simulink model "TVCLaunch"  (R2024b)
settings: Solver=VariableStepAuto  StartTime=0.0  StopTime=30  FixedStep=0.0001  MaxStep=0.0001  RelTol=1e-3
model workspace (MAT data in the model file):
  Mass = 0.5
undefined symbols (not defined in the file): DiscIntNeverNeededParam
libraries: simulink x3, simulink_extras x2, slpidlib x2, dspfdesign x1
settings Model: Creator=jebid  LastModifiedBy=jebid

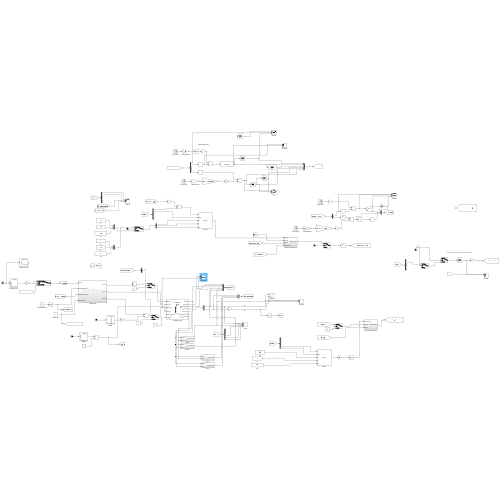
[thumbnail: Simulink's stored preview of the top-level diagram]
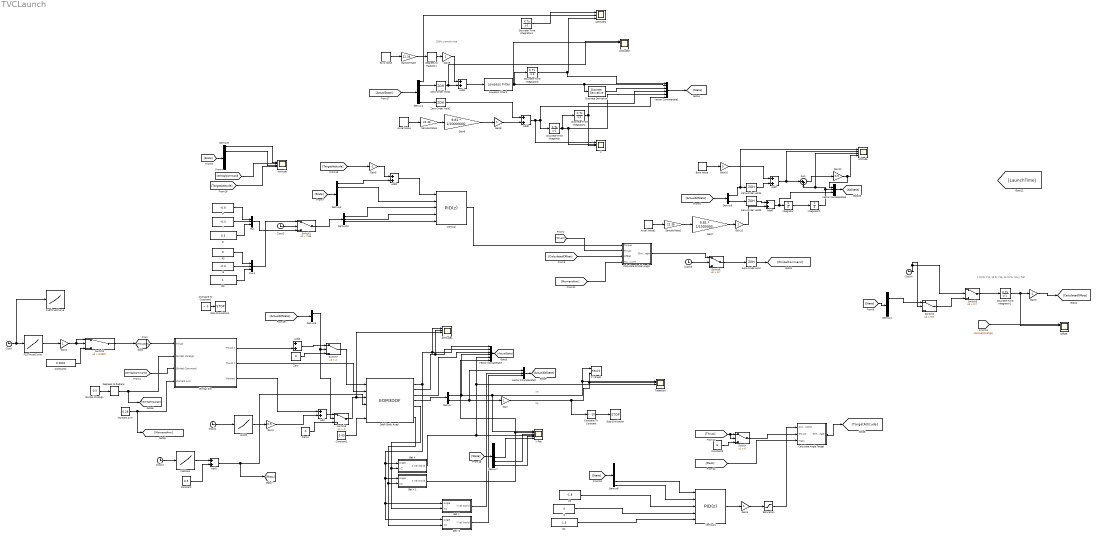
== system TVCLaunch ==
  note: 250hz sample rate
  note: 1.19 for F10, 18 for F15, 23.75 for noisy f15?
  note: Ze
  note: Xe
  3dof (Body Axes) : EOM3DOF  mtype=Custom Variable  v_ini=0  theta_ini=0.09  mass=0.5  Iyy=0.05  g=-9.81  abi_flag=on
  Accel Noise : RandomNumber  Variance=70  SampleTime=0.002
  Accel Noise1 : RandomNumber  Variance=70  SampleTime=0.002
  Add{,1..7} (8 alike) : Sum
  Altitude : Scope  NumInputPorts=5
  Attitude{,1..2,4} (4 alike) : Scope  NumInputPorts=5
  BUMP : Lookup_n-D  NumberOfTableDimensions=1  BreakpointsForDimension1=[-5 -4 -3 -2 -1 0 1 1.1000000000000001 1.2 1.3 5]  Table=[0 0 0 0 0 0 0 0.28000000000000003 0.28000000000000003 0 0]  InternalRulePriority=Speed  RndMeth=Simplest
  Baro Noise : RandomNumber  Variance=0.1  SampleTime=0.002
  Calculate Angle Target : Subsystem
  Calculate Gimbal Angle : Subsystem
  Clock{,1..2,4..6} (6 alike) : Clock
  Compare To Constant : simulink/Logic and Bit Operations/Compare To Constant  relop=<  const=-10  OutDataTypeStr=boolean
  Compare To Constant1 : simulink/Logic and Bit Operations/Compare To Constant  relop=<  const=0  OutDataTypeStr=boolean
  Constant : Constant  Value=0.5
  Constant1 : Constant  Value=0.05
  Constant2 : Constant  Value=0.0001
  Constant3 : Constant  Value=6
  D : Constant  Value=0.3
  D2 : Constant  Value=1.5
  D3 : Constant
  Degrees to Radians : simulink_extras/Transformations/Degrees to Radians
  Degrees to Radians1 : simulink_extras/Transformations/Degrees to Radians
  Demux : Demux  Outputs=2
  Demux{1,3..7} (6 alike) : Demux  Outputs=6
  Demux10 : Demux  Outputs=3
  Demux8 : Demux  Outputs=3
  Demux9 : Demux  Outputs=3
  Discrete Derivative : simulink/Discrete/Discrete Derivative  gainval=1.0  ICPrevScaledInput=0.0  OutMin=[]  OutMax=[]  OutDataType=fixdt(1, 16)  OutScaling=2^-10  DoSatur=off
  Discrete-Time Integrator : DiscreteIntegrator  SampleTime=0.01  ICPrevOutput=DiscIntNeverNeededParam  ICPrevScaledInput=DiscIntNeverNeededParam
  Discrete-Time Integrator1 : DiscreteIntegrator  gainval=20  SampleTime=0.01  ICPrevOutput=DiscIntNeverNeededParam  ICPrevScaledInput=DiscIntNeverNeededParam
  Discrete-Time Integrator2 : DiscreteIntegrator  SampleTime=0.01  ICPrevOutput=DiscIntNeverNeededParam  ICPrevScaledInput=DiscIntNeverNeededParam
  Discrete-Time Integrator3 : DiscreteIntegrator  InitialCondition=0.09  SampleTime=0.01  ICPrevOutput=DiscIntNeverNeededParam  ICPrevScaledInput=DiscIntNeverNeededParam
  Discrete-Time Integrator4 : DiscreteIntegrator  SampleTime=0.01  ICPrevOutput=DiscIntNeverNeededParam  ICPrevScaledInput=DiscIntNeverNeededParam
  F10ThrustCurve : Lookup_n-D  NumberOfTableDimensions=1  BreakpointsForDimension1=[0.015;0.077;0.201;0.31;0.464;0.573;0.789;1.068;1.393;1.718;2.166;2.677;3.311;3.683;3.791;4.101;4.658;5.168;5.725;6.112;6.329;6.499;6.685;6.778;6.917;7.025;7.13]  Table=[28.22;26.082;24.934;22.806;20.183;17.886;16.075;13.946;12.63;11.155;9.843999999999999;9.515000000000001;9.186999999999999;8.859;9.679;9.679;9.515000000000001;9.023;9.023;8.531000000000001;8.859;7.546;5.742;4.921;2.625;1.312;-0.001]  InternalRulePriority=Speed  RndMeth=Simplest
  F15Mass : Lookup_n-D  NumberOfTableDimensions=1  BreakpointsForDimension1=[0;0.14799999999999999;0.22800000000000001;0.29399999999999998;0.35299999999999998;0.38200000000000001;0.41899999999999998;0.47699999999999998;0.52000000000000002;0.59299999999999997;0.68799999999999994;0.85499999999999998;1.0369999999999999;1.2050000000000001;1.423;1.452;1.5029999999999999;1.736;1.9550000000000001;2.21;2.4940000000000002;2.7629999999999999;3.1200000000000001;3.3820000000000001;3.4039999999999999;3.4180000000000001;3.4500000000000002;60]  Table=[0.102;0.101316;0.100354;0.09921099999999999;0.09790500000000001;0.097151;0.096077;0.09438199999999999;0.09324;0.091477;0.089374;0.085969;0.082485;0.079399;0.0755;0.07496700000000001;0.07402599999999999;0.069882;0.066051;0.061665;0.056863;0.052445;0.046687;0.042513;0.042215;0.042095;0.042;0.042]  InternalRulePriority=Speed  RndMeth=Simplest
  F15ThrustCurve : Lookup_n-D  NumberOfTableDimensions=1  BreakpointsForDimension1=[0;0.14799999999999999;0.22800000000000001;0.29399999999999998;0.35299999999999998;0.38200000000000001;0.41899999999999998;0.47699999999999998;0.52000000000000002;0.59299999999999997;0.68799999999999994;0.85499999999999998;1.0369999999999999;1.2050000000000001;1.423;1.452;1.5029999999999999;1.736;1.9550000000000001;2.21;2.4940000000000002;2.7629999999999999;3.1200000000000001;3.3820000000000001;3.4039999999999999;3.4180000000000001;3.4500000000000002;60]  Table=[0;7.6379999999999999;12.253;16.390999999999998;20.210000000000001;22.756;25.260000000000002;23.074000000000002;20.844999999999999;19.093;17.5;16.225000000000001;15.427;14.948;14.627000000000001;15.741;14.785;14.622999999999999;14.303000000000001;14.141;13.819000000000001;13.337999999999999;13.334;13.013;9.3520000000000003;4.8949999999999996;-0.001;-0.001]  InternalRulePriority=Speed  RndMeth=Simplest
  Gain{,2,4,8..9,11} (6 alike) : Gain
  Gain1 : Gain  Gain=0.5
  Gain10 : Gain  Gain=5
  Gain12 : Gain  Gain=0.5
  Gain3 : Gain  Gain=-1
  Gain5 : Gain  Gain=-1
  Gain6 : Gain  Gain=9.81 * 1/10000000
  Gain7 : Gain  Gain=9.81 * 1/1000000
  Get X : Subsystem
  Get X 1 : Subsystem
  Get Y : Subsystem
  Get Y1 : Subsystem
  Gimbal Misalign : Constant  Value=0.5
  Gimbal Sim : Subsystem
  Gyro Noise : RandomNumber  Variance=0.0028  SampleTime=0.002
  I : Constant  Value=-0.3  VectorParams1D=off
  I2 : Constant  Value=0  VectorParams1D=off
  I3 : Constant  Value=-0.3  VectorParams1D=off
  Integrator : Integrator
  Integrator1 : Integrator
  Lowpass Filter1 : dspfdesign/Lowpass Filter  FilterType=IIR  DesignForMinimumOrder=on  FilterOrder=50  PassbandFrequency=7.5  StopbandFrequency=247.5  PassbandRipple=0.1  StopbandAttenuation=100  SampleRateMode=Specify on dialog  SampleRate=500  SimulateUsing=Interpreted execution  roundingMode=Floor  coeffsDataTypeStr=fixdt(1,16)
  Moment Arm : Constant  Value=0.28
  Mux : Mux  Inputs=3
  Mux1 : Mux  Inputs=3
  Offset : Scope  NumInputPorts=5
  P : Constant  Value=-0.9
  P2 : Constant  Value=-1.8
  P3 : Constant  Value=0
  Sample Rate : Gain  Gain=22.36
  Sample Rate1 : Gain  Gain=22.36
  Sample Rate2 : Gain  Gain=22.36
  Saturation : Saturate  UpperLimit=8  LowerLimit=-8
  Stop Simulation : Stop
  Stop Simulation1 : Stop
  Sum : Sum  Inputs=|++
  Switch : Switch  Criteria=u2 > Threshold  Threshold=6  SaturateOnIntegerOverflow=off  InputSameDT=off
  Switch1 : Switch  Criteria=u2 > Threshold  Threshold=2.85  SaturateOnIntegerOverflow=off  InputSameDT=off
  Switch2 : Switch  Criteria=u2 > Threshold  Threshold=0.6  SaturateOnIntegerOverflow=off  InputSameDT=off
  Switch3 : Switch  Criteria=u2 > Threshold  Threshold=0.7  SaturateOnIntegerOverflow=off  InputSameDT=off
  Switch4 : Switch  Criteria=u2 > Threshold  Threshold=0.0001  SaturateOnIntegerOverflow=off  InputSameDT=off
  Switch6 : Switch  Criteria=u2 > Threshold  Threshold=0.7  SaturateOnIntegerOverflow=off  InputSameDT=off
  Switch7 : Switch  Criteria=u2 > Threshold  Threshold=2  SaturateOnIntegerOverflow=off  InputSameDT=off
  Switch8 : Switch  Criteria=u2 > Threshold  Threshold=2  SaturateOnIntegerOverflow=off  InputSameDT=off
  Trajectory : Scope  NumInputPorts=5
  Vector Concatenate : Concatenate  NumInputs=6
  Vector Concatenate1 : Concatenate  NumInputs=6
  Vector Concatenate2 : Concatenate  NumInputs=3
  Vector Concatenate3 : Concatenate  NumInputs=3
  Vertical : slpidlib/PID Controller  Controller=PID  Form=Parallel  TimeDomain=Discrete-time  UseExternalTs=off  SampleTime=0.01  IntegratorMethod=Forward Euler  FilterMethod=Forward Euler  ControllerParametersSource=external  P=1  I=1  UseKiTs=off  D=0  UseExternalDerivativeSource=on  N=100  UseFilter=off  TunerSelectOption=Transfer Function Based (PID Tuner App)  InitialConditionSource=internal  InitialConditionForIntegrator=0  InitialConditionForFilter=0  DifferentiatorICPrevScaledInput=0  ExternalReset=none  TrackingMode=off  Kt=1  LimitOutput=off  SatLimitsSource=internal  UpperSaturationLimit=inf  LowerSaturationLimit=-inf  LinearizeAsGain=off  AntiWindupMode=none  Kb=1  LimitIntegrator=off  UpperIntegratorSaturationLimit=inf  LowerIntegratorSaturationLimit=-inf  POutMin=[]  POutMax=[]  IOutMin=[]  IOutMax=[]  DOutMin=[]  DOutMax=[]  NOutMin=[]  NOutMax=[]  SumOutMin=[]  SumOutMax=[]  SaturationOutMin=[]  SaturationOutMax=[]  PParamMin=[]  PParamMax=[]  IParamMin=[]  IParamMax=[]  DParamMin=[]  DParamMax=[]  NParamMin=[]  NParamMax=[]  KbParamMin=[]  KbParamMax=[]  KtParamMin=[]  KtParamMax=[]  KbOutMin=[]  KbOutMax=[]  KtOutMin=[]  KtOutMax=[]  IntegratorOutMin=[]  IntegratorOutMax=[]  FilterOutMin=[]  FilterOutMax=[]  SumI1OutMin=[]  SumI1OutMax=[]  SumI2OutMin=[]  SumI2OutMax=[]  SumI3OutMin=[]  SumI3OutMax=[]  SumI4OutMin=[]  SumI4OutMax=[]  SumDOutMin=[]  SumDOutMax=[]  DifferentiatorOutMin=[]  DifferentiatorOutMax=[]  FilterDiffOutCoefMin=[]  FilterDiffOutCoefMax=[]  ReciprocalOutMin=[]  ReciprocalOutMax=[]  SumDenOutMin=[]  SumDenOutMax=[]  SumNumOutMin=[]  SumNumOutMax=[]  DivideOutMin=[]  DivideOutMax=[]  UdiffTsProdOutMin=[]  UdiffTsProdOutMax=[]  NTsProdOutMin=[]  NTsProdOutMax=[]  UintegralTsProdOutMin=[]  UintegralTsProdOutMax=[]  UngainTsProdOutMin=[]  UngainTsProdOutMax=[]  ClampingZeroOutDataTypeStr=Inherit: Inherit via back propagation  ClampingZeroOutMin=[]  ClampingZeroOutMax=[]  FilterDenConstantOutDataTypeStr=Inherit: Inherit via back propagation  FilterDenConstantOutMin=[]  FilterDenConstantOutMax=[]  PCopyOutDataTypeStr=Inherit: Inherit via back propagation  PCopyOutMin=[]  PCopyOutMax=[]  NCopyOutDataTypeStr=Inherit: Inherit via back propagation  NCopyOutMin=[]  NCopyOutMax=[]  IntegratorContinuousStateAttributes=''  IntegratorStateMustResolveToSignalObject=off  IntegratorRTWStateStorageClass=Auto  FilterContinuousStateAttributes=''  FilterStateMustResolveToSignalObject=off  FilterRTWStateStorageClass=Auto  ParallelPVariant=ExternalParameters  IdealPVariant=Disabled  IVariant=ExternalParameters  DVariant=ExternalParameters  IntegratorVariant=Discrete  SatVariant=Disabled  AWVariant=Passthrough  PCopyVariant=Disabled  TRVariant=Disabled  FdbkBlocksVariant=Forward  IdealPFdbkVariant=Disabled  SatFdbkVariant=Disabled  DerivativeFilterVariant=Passthrough  NVariant=Passthrough  NCopyVariant=Disabled_SignalSpec  FilterICVariant=Disabled  IntegratorICVariant=InternalICs  ExternalResetVariant=Disabled  TRSumVariant=Passthrough  SumFdbkVariant=Disabled  SumVariant=Sum_PID  TsampFilterVariant=InternalTs  TsampNgainVariant=Passthrough  TsampIntegralVariant=Disabled_SignalSpec  ExternalSaturationOutDataTypeStr=Inherit: Same as second input  DerivativeSourceVariant=ExternalYdot  PreIntVariant=InternalPreInt
      settings: LibrarySourceBlock=simulink/Discrete/Discrete PID Controller
  Vertical1 : slpidlib/PID Controller  Controller=PID  Form=Parallel  TimeDomain=Discrete-time  UseExternalTs=off  SampleTime=0.01  IntegratorMethod=Forward Euler  FilterMethod=Forward Euler  ControllerParametersSource=external  P=1  I=1  UseKiTs=off  D=0  UseExternalDerivativeSource=on  N=100  UseFilter=off  TunerSelectOption=Transfer Function Based (PID Tuner App)  InitialConditionSource=internal  InitialConditionForIntegrator=0  InitialConditionForFilter=0  DifferentiatorICPrevScaledInput=0  ExternalReset=none  TrackingMode=off  Kt=1  LimitOutput=off  SatLimitsSource=internal  UpperSaturationLimit=inf  LowerSaturationLimit=-inf  LinearizeAsGain=off  AntiWindupMode=none  Kb=1  LimitIntegrator=off  UpperIntegratorSaturationLimit=inf  LowerIntegratorSaturationLimit=-inf  POutMin=[]  POutMax=[]  IOutMin=[]  IOutMax=[]  DOutMin=[]  DOutMax=[]  NOutMin=[]  NOutMax=[]  SumOutMin=[]  SumOutMax=[]  SaturationOutMin=[]  SaturationOutMax=[]  PParamMin=[]  PParamMax=[]  IParamMin=[]  IParamMax=[]  DParamMin=[]  DParamMax=[]  NParamMin=[]  NParamMax=[]  KbParamMin=[]  KbParamMax=[]  KtParamMin=[]  KtParamMax=[]  KbOutMin=[]  KbOutMax=[]  KtOutMin=[]  KtOutMax=[]  IntegratorOutMin=[]  IntegratorOutMax=[]  FilterOutMin=[]  FilterOutMax=[]  SumI1OutMin=[]  SumI1OutMax=[]  SumI2OutMin=[]  SumI2OutMax=[]  SumI3OutMin=[]  SumI3OutMax=[]  SumI4OutMin=[]  SumI4OutMax=[]  SumDOutMin=[]  SumDOutMax=[]  DifferentiatorOutMin=[]  DifferentiatorOutMax=[]  FilterDiffOutCoefMin=[]  FilterDiffOutCoefMax=[]  ReciprocalOutMin=[]  ReciprocalOutMax=[]  SumDenOutMin=[]  SumDenOutMax=[]  SumNumOutMin=[]  SumNumOutMax=[]  DivideOutMin=[]  DivideOutMax=[]  UdiffTsProdOutMin=[]  UdiffTsProdOutMax=[]  NTsProdOutMin=[]  NTsProdOutMax=[]  UintegralTsProdOutMin=[]  UintegralTsProdOutMax=[]  UngainTsProdOutMin=[]  UngainTsProdOutMax=[]  ClampingZeroOutDataTypeStr=Inherit: Inherit via back propagation  ClampingZeroOutMin=[]  ClampingZeroOutMax=[]  FilterDenConstantOutDataTypeStr=Inherit: Inherit via back propagation  FilterDenConstantOutMin=[]  FilterDenConstantOutMax=[]  PCopyOutDataTypeStr=Inherit: Inherit via back propagation  PCopyOutMin=[]  PCopyOutMax=[]  NCopyOutDataTypeStr=Inherit: Inherit via back propagation  NCopyOutMin=[]  NCopyOutMax=[]  IntegratorContinuousStateAttributes=''  IntegratorStateMustResolveToSignalObject=off  IntegratorRTWStateStorageClass=Auto  FilterContinuousStateAttributes=''  FilterStateMustResolveToSignalObject=off  FilterRTWStateStorageClass=Auto  ParallelPVariant=ExternalParameters  IdealPVariant=Disabled  IVariant=ExternalParameters  DVariant=ExternalParameters  IntegratorVariant=Discrete  SatVariant=Disabled  AWVariant=Passthrough  PCopyVariant=Disabled  TRVariant=Disabled  FdbkBlocksVariant=Forward  IdealPFdbkVariant=Disabled  SatFdbkVariant=Disabled  DerivativeFilterVariant=Passthrough  NVariant=Passthrough  NCopyVariant=Disabled_SignalSpec  FilterICVariant=Disabled  IntegratorICVariant=InternalICs  ExternalResetVariant=Disabled  TRSumVariant=Passthrough  SumFdbkVariant=Disabled  SumVariant=Sum_PID  TsampFilterVariant=InternalTs  TsampNgainVariant=Passthrough  TsampIntegralVariant=Disabled_SignalSpec  ExternalSaturationOutDataTypeStr=Inherit: Same as second input  DerivativeSourceVariant=ExternalYdot  PreIntVariant=InternalPreInt
      settings: LibrarySourceBlock=simulink/Discrete/Discrete PID Controller
  X : Scope  NumInputPorts=5
  X Pos : Scope  NumInputPorts=6
  XY Graph : Record  FileSettingsInternal="{\"entries\":[{\"content\":{\"excelSettings\":{\"content\":{},\"type\":\"Streamout.ExcelSettings\"}},\"type\":\"Streamout.FileSettingStorage\",\"uuid\":\"\"}],\"packageUris\":[\"http:\\/\\/schema.mathworks.com\\/mf0\\/streamout_blocks\\/R2020a\"],\"version\":\"1.0\"}"  Layout=[1 1]  SignalsInternal="{\"entries\":[{\"content\":{\"signals\":[{\"content\":{\"blockPath\":[],\"dimensions\":[1],\"domain\":\"\",\"lineColor\":\"#a2142f\",\"plots\":[ 1 ],\"port\":1,\"sid\":[\"\"],\"signalID\":1,\"signalName\":\"Demux:1\"},\"type\":\"RecordBlkView.Signal\",\"uuid\":\"\"},{\"content\":{\"blockPath\":[],\"dimensions\":[1],\"domain\":\"\",\"lineColor\":\"#139fff\",\"plots\":[ 1 ],\"port\":2,\"sid\":[\"\"],\"signalID\":2,\"signalName\":\"Gain\"},\"type\":\"RecordBlkView.Signal\",\"uuid\":\"\"}]},\"type\":\"RecordBlkView.InputSignals\",\"uuid\":\"\"}],\"packageUris\":[\"http:\\/\\/schema.mathworks.com\\/mf0\\/streamout_blocks\\/R2020a\"],\"version\":\"1.0\"}"  VisualizationBindings="{\"xyplotplugin\":{\"info\":[{\"series\":[{\"bindingParametersList\":[{\"parameter\":\"X-Axis\",\"signalID\":1,\"signalName\":\"Demux:1\"},{\"parameter\":\"Y-Axis\",\"signalID\":2,\"signalName\":\"Gain\"}],\"seriesID\":0}],\"subplotID\":1}]}}"  CompatibilityTag=XY
  Zero : Constant  Value=0  OutDataTypeStr=Inherit: Inherit via back propagation
  Zero-Order Hold : ZeroOrderHold  SampleTime=0.02
  Zero-Order Hold{1..4} (4 alike) : ZeroOrderHold  SampleTime=0.002
  Zero1 : Constant  Value=0  OutDataTypeStr=Inherit: Inherit via back propagation
  wires:
  3dof (Body Axes)/4 -> Demux/1
  Demux/2 -> Vector Concatenate2/1, Gain/1
  Gain/1 -> Compare To Constant/1, XY Graph/2, Trajectory/2
  Clock/1 -> F10ThrustCurve/1, F15ThrustCurve/1
  Compare To Constant/1 -> Stop Simulation/1
  Gimbal Misalign/1 -> Degrees to Radians/1
  Moment Arm/1 -> [MomentArm], Gimbal Sim/4(Moment Arm)
  3dof (Body Axes)/1 -> Get Y1/1(Angle), Get Y/1(Angle), Get X 1/1(Angle), Get X/1(Angle), Attitude4/1, Vector Concatenate/1
  3dof (Body Axes)/2 -> Attitude4/2, Vector Concatenate/2
  Clock1/1 -> BUMP/1
  Degrees to Radians/1 -> [GimbalMisalign], Gimbal Sim/2(Gimbal Misalign)
  Gimbal Sim/2(Thurst Z) -> 3dof (Body Axes)/2
  Gimbal Sim/1(Thrust X) -> Add3/2
  Compare To Constant1/1 -> Stop Simulation1/1
  Constant2/1 -> Switch4/3
  Gimbal Sim/3(Moment) -> Add/1
  BUMP/1 -> Gain1/1
  Gain1/1 -> Add/2
  3dof (Body Axes)/3 -> Vector Concatenate/3
  Clock4/1 -> Switch2/2, Switch3/2
  Switch3/1 -> Discrete-Time Integrator1/1
  Switch4/1 -> [Thrust]
  [Thrust] -> Gimbal Sim/1(Thrust)
  Clock6/1 -> Switch6/2
  Switch6/1 -> Zero-Order Hold/1
  Zero-Order Hold/1 -> [GimbalCommand]
  [CalculatedOffset] -> Calculate Gimbal Angle/3(Offset)
  Vertical/1 -> Calculate Gimbal Angle/1(Torque)
  [GimbalCommand] -> Gimbal Sim/3(Gimbal Command)
  [GimbalCommand] -> Attitude/2
  Vector Concatenate/1 -> [ActualState]
  [State] -> Demux3/1
  Demux3/2 -> Vertical/2
  [State] -> Demux4/1
  [State] -> Demux5/1
  Demux5/1 -> Attitude/1
  Demux5/2 -> Attitude/3
  P2/1 -> Vertical1/3
  D2/1 -> Vertical1/5
  I2/1 -> Vertical1/4
  [State] -> Demux6/1
  [Thrust] -> Calculate Gimbal Angle/2(Thrust)
  [MomentArm] -> Calculate Gimbal Angle/4(Moment Arm)
  Calculate Gimbal Angle/1(Gimbal Angle) -> Switch6/1
  Gain2/1 -> Switch4/1, Switch4/2
  Discrete-Time Integrator1/1 -> Offset/2, Gain3/1
  [GimbalMisalign] -> Offset/1
  Clock2/1 -> F15Mass/1
  F15Mass/1 -> Add1/1
  Add1/1 -> [Mass], 3dof (Body Axes)/4
  Constant/1 -> Add1/2
  Constant1/1 -> 3dof (Body Axes)/6
  Vertical1/1 -> Gain4/1
  [Mass] -> Calculate Angle Target/3(Mass)
  Add2/1 -> Vertical/1
  Demux3/1 -> Add2/2
  Gain4/1 -> Saturation/1
  [TargetAttitude] -> Gain5/1
  Gain5/1 -> Add2/1
  Demux6/5 -> Vertical1/1
  Demux6/6 -> Vertical1/2
  [TargetAttitude] -> Attitude/4
  Add3/1 -> Switch7/1
  F15ThrustCurve/1 -> Gain2/1
  Vector Concatenate1/1 -> [State]
  [ActualState] -> Demux1/1
  Saturation/1 -> Calculate Angle Target/1(Acceleration)
  Switch/1 -> Calculate Angle Target/2(Thrust)
  [Thrust] -> Switch/2, Switch/1
  Constant3/1 -> Switch/3
  Demux1/2 -> Zero-Order Hold1/1
  Gyro Noise/1 -> Sample Rate/1
  Zero-Order Hold1/1 -> Attitude2/1, Add4/2
  Degrees to Radians1/1 -> Gain9/1
  Demux1/6 -> Zero-Order Hold2/1
  Zero-Order Hold2/1 -> Add5/1
  Gain6/1 -> Gain8/1
  Accel Noise/1 -> Sample Rate1/1
  Add5/1 -> X/1, Discrete-Time Integrator/1, Vector Concatenate1/6
  Discrete-Time Integrator3/1 -> Attitude1/5, Vector Concatenate1/1
  Discrete-Time Integrator2/1 -> X/3, Vector Concatenate1/4
  Discrete-Time Integrator/1 -> Discrete-Time Integrator2/1, X/2, Vector Concatenate1/5
  Discrete Derivative/1 -> Vector Concatenate1/3
  Get X/1(X Vel World) -> Trajectory/3, Vector Concatenate/5, X Pos/4
  Get X 1/1(X Vel World) -> X Pos/2, Vector Concatenate/6
  Demux/1 -> Vector Concatenate/4, X Pos/1, XY Graph/1, Trajectory/1
  3dof (Body Axes)/5 -> Get Y/2(XZ), Get X/2(XZ)
  3dof (Body Axes)/7 -> Get Y1/2(XZ), Get X 1/2(XZ)
  [State] -> Demux7/1
  Demux7/6 -> X Pos/5
  Demux7/5 -> X Pos/3
  Demux7/4 -> X Pos/6
  Vector Concatenate2/1 -> [ActualAltState]
  Get Y1/1(Y Vel World) -> Vector Concatenate2/3
  Get Y/1(Y Vel World) -> Vector Concatenate2/2
  Vector Concatenate3/1 -> [AltState]
  Gain7/1 -> Gain11/1
  Zero-Order Hold3/1 -> Add6/1
  [ActualAltState] -> Demux8/1
  Demux8/3 -> Zero-Order Hold3/1
  Demux8/1 -> Altitude/1, Zero-Order Hold4/1
  Baro Noise/1 -> Gain10/1
  Zero-Order Hold4/1 -> Add7/2
  Add7/1 -> Sum/1, Altitude/2
  Gain8/1 -> Add5/2
  Gain9/1 -> Add4/1
  Gain10/1 -> Add7/1
  Gain11/1 -> Add6/2
  Sample Rate/1 -> Degrees to Radians1/1
  Sample Rate1/1 -> Gain6/1
  Sample Rate2/1 -> Gain7/1
  Add4/1 -> Lowpass Filter1/1
  Accel Noise1/1 -> Sample Rate2/1
  Add6/1 -> Vector Concatenate3/3, Integrator/1
  Integrator/1 -> Integrator1/1
  Integrator1/1 -> Vector Concatenate3/2, Sum/2, Altitude/4
  Sum/1 -> Gain12/1
  Gain12/1 -> Vector Concatenate3/1, Altitude/5
  Lowpass Filter1/1 -> Attitude2/2, Vector Concatenate1/2, Discrete Derivative/1, Discrete-Time Integrator3/1
  Calculate Angle Target/1(Gimbal Angle) -> [TargetAttitude]
  Discrete-Time Integrator4/1 -> Attitude1/1
  Demux1/1 -> Attitude1/3
  Switch2/1 -> Switch3/3
  Switch7/1 -> 3dof (Body Axes)/1
  Add/1 -> Switch8/1
  Switch8/1 -> Attitude4/4, 3dof (Body Axes)/3
  Demux4/2 -> Switch2/1
  [ActualAltState] -> Demux9/1
  Demux9/1 -> Switch8/2, Switch7/2
  Zero/1 -> Switch7/3
  Zero1/1 -> Switch8/3
  I/1 -> Mux/2
  P/1 -> Mux/1
  D/1 -> Mux/3
  Demux10/2 -> Vertical/4
  Demux10/3 -> Vertical/5
  Demux10/1 -> Vertical/3
  D3/1 -> Mux1/3
  P3/1 -> Mux1/1
  I3/1 -> Mux1/2
  Clock5/1 -> Switch1/2
  Mux1/1 -> Switch1/1
  Mux/1 -> Switch1/3
  Switch1/1 -> Demux10/1
  Gain3/1 -> [CalculatedOffset]

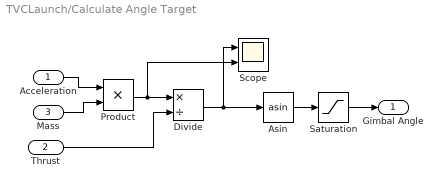
== system TVCLaunch/Calculate Angle Target ==
  Acceleration : Inport
  Thrust : Inport  Port=2
  Mass : Inport  Port=3
  Asin : Trigonometry  Operator=asin
  Divide : Product  Inputs=*/
  Product : Product
  Saturation : Saturate  UpperLimit=0.4  LowerLimit=-0.4
  Scope : Scope  NumInputPorts=2
  Gimbal Angle : Outport
  wires:
  Asin/1 -> Saturation/1
  Acceleration/1 -> Product/1
  Mass/1 -> Product/2
  Product/1 -> Scope/2, Divide/1
  Thrust/1 -> Divide/2
  Divide/1 -> Scope/1, Asin/1
  Saturation/1 -> Gimbal Angle/1

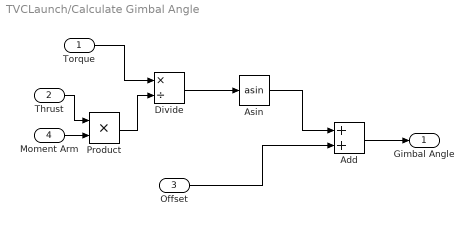
== system TVCLaunch/Calculate Gimbal Angle ==
  Torque : Inport
  Thrust : Inport  Port=2
  Offset : Inport  Port=3
  Moment Arm : Inport  Port=4
  Add : Sum
  Asin : Trigonometry  Operator=asin
  Divide : Product  Inputs=*/
  Product : Product
  Gimbal Angle : Outport
  wires:
  Add/1 -> Gimbal Angle/1
  Offset/1 -> Add/2
  Moment Arm/1 -> Product/2
  Thrust/1 -> Product/1
  Torque/1 -> Divide/1
  Product/1 -> Divide/2
  Divide/1 -> Asin/1
  Asin/1 -> Add/1

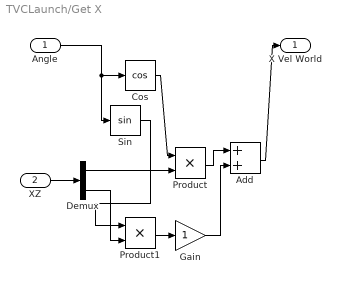
== system TVCLaunch/Get X ==
  Angle : Inport
  XZ : Inport  Port=2
  Add : Sum
  Cos : Trigonometry  Operator=cos
  Demux : Demux  Outputs=2
  Gain : Gain
  Product : Product
  Product1 : Product
  Sin : Trigonometry
  X Vel World : Outport
  wires:
  Angle/1 -> Sin/1, Cos/1
  XZ/1 -> Demux/1
  Add/1 -> X Vel World/1
  Cos/1 -> Product/1
  Sin/1 -> Product1/1
  Product/1 -> Add/1
  Product1/1 -> Gain/1
  Gain/1 -> Add/2
  Demux/2 -> Product1/2
  Demux/1 -> Product/2

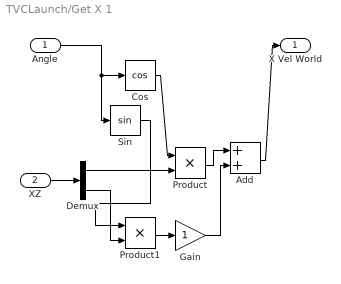
== system TVCLaunch/Get X 1 ==
  Angle : Inport
  XZ : Inport  Port=2
  Add : Sum
  Cos : Trigonometry  Operator=cos
  Demux : Demux  Outputs=2
  Gain : Gain
  Product : Product
  Product1 : Product
  Sin : Trigonometry
  X Vel World : Outport
  wires:
  Angle/1 -> Sin/1, Cos/1
  XZ/1 -> Demux/1
  Add/1 -> X Vel World/1
  Cos/1 -> Product/1
  Sin/1 -> Product1/1
  Product/1 -> Add/1
  Product1/1 -> Gain/1
  Gain/1 -> Add/2
  Demux/2 -> Product1/2
  Demux/1 -> Product/2

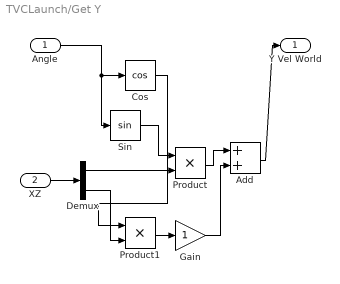
== system TVCLaunch/Get Y ==
  Angle : Inport
  XZ : Inport  Port=2
  Add : Sum
  Cos : Trigonometry  Operator=cos
  Demux : Demux  Outputs=2
  Gain : Gain
  Product : Product
  Product1 : Product
  Sin : Trigonometry
  Y Vel World : Outport
  wires:
  Angle/1 -> Sin/1, Cos/1
  XZ/1 -> Demux/1
  Add/1 -> Y Vel World/1
  Product/1 -> Add/1
  Product1/1 -> Gain/1
  Gain/1 -> Add/2
  Demux/2 -> Product1/2
  Demux/1 -> Product/2
  Sin/1 -> Product/1
  Cos/1 -> Product1/1

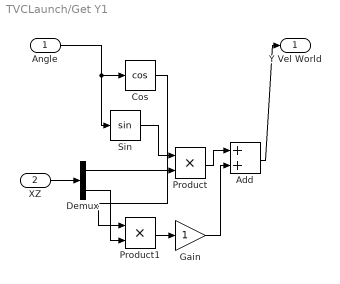
== system TVCLaunch/Get Y1 ==
  Angle : Inport
  XZ : Inport  Port=2
  Add : Sum
  Cos : Trigonometry  Operator=cos
  Demux : Demux  Outputs=2
  Gain : Gain
  Product : Product
  Product1 : Product
  Sin : Trigonometry
  Y Vel World : Outport
  wires:
  Angle/1 -> Sin/1, Cos/1
  XZ/1 -> Demux/1
  Add/1 -> Y Vel World/1
  Product/1 -> Add/1
  Product1/1 -> Gain/1
  Gain/1 -> Add/2
  Demux/2 -> Product1/2
  Demux/1 -> Product/2
  Sin/1 -> Product/1
  Cos/1 -> Product1/1

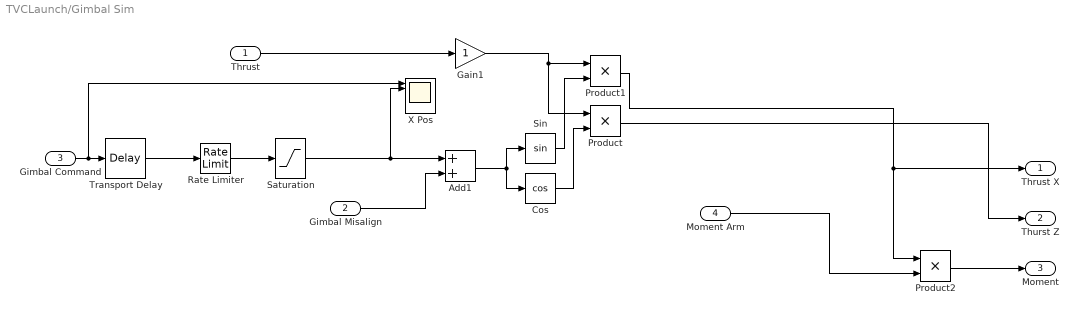
== system TVCLaunch/Gimbal Sim ==
  Thrust : Inport
  Gimbal Misalign : Inport  Port=2
  Gimbal Command : Inport  Port=3
  Moment Arm : Inport  Port=4
  Add1 : Sum
  Cos : Trigonometry  Operator=cos
  Gain1 : Gain
  Product : Product
  Product1 : Product
  Product2 : Product
  Rate Limiter : RateLimiter  RisingSlewLimit=0.9  FallingSlewLimit=-0.9
  Saturation : Saturate  UpperLimit=0.0872665  LowerLimit=-0.0872665
  Sin : Trigonometry
  Transport Delay : TransportDelay  DelayTime=0.03
  X Pos : Scope  NumInputPorts=6
  Thrust X : Outport
  Thurst Z : Outport  Port=2
  Moment : Outport  Port=3
  wires:
  Thrust/1 -> Gain1/1
  Product1/1 -> Thrust X/1, Product2/1
  Gain1/1 -> Product1/1, Product/1
  Product/1 -> Thurst Z/1
  Moment Arm/1 -> Product2/2
  Cos/1 -> Product/2
  Sin/1 -> Product1/2
  Add1/1 -> Cos/1, Sin/1
  Gimbal Misalign/1 -> Add1/2
  Product2/1 -> Moment/1
  Gimbal Command/1 -> X Pos/1, Transport Delay/1
  Transport Delay/1 -> Rate Limiter/1
  Rate Limiter/1 -> Saturation/1
  Saturation/1 -> X Pos/2, Add1/1
